simulink model "conicaltank"  (R2021a)
settings: Solver=ode45  StartTime=0.0  StopTime=30  RelTol=1e-3  EnableMultiTasking=on
settings Model: Creator=Administrator  LastModifiedBy=rakhul
settings SolverCC: AlgebraicLoopSolver=TrustRegion
settings DataIOCC: ExternalInput=[0 111.111]  InitialState=[]  LimitDataPoints=on  LoadExternalInput=on  LoadInitialState=on  SaveFormat=Array  ReturnWorkspaceOutputs=off
settings OptimizationCC: DefaultParameterBehavior=Inlined  BufferReuse=off  LifeSpan=inf
settings DebuggingCC: UnderspecifiedInitializationDetection=Classic  MergeDetectMultiDrivingBlocksExec=none  SolverPrmCheckMsg=warning  StateNameClashWarn=warning  InitInArrayFormatMsg=none  SFUnexpectedBacktrackingDiag=warning  SFNoUnconditionalDefaultTransitionDiag=warning  SFExecutionAtInitializationDiag=none  SFMachineParentedDataDiag=warning  ArithmeticOperatorsInVariantConditions=warning
settings HardwareCC: ProdBitPerPointer=32  ProdBitPerSizeT=32  ProdBitPerPtrDiffT=32  ProdLargestAtomicFloat=None  ProdIntDivRoundTo=Undefined  ProdEndianess=Unspecified  ProdWordSize=32  ProdHWDeviceType=32-bit Generic
settings ModelReferenceCC: PropagateSignalLabelsOutOfModel=off
settings SFSimCC: SimUseLocalCustomCode=off  CustomCodeUndefinedFunction=UseInterfaceOnly
settings RTWCC: RTWUseLocalCustomCode=off
settings CodeAppCC: StateflowObjectComments=on
settings GRTTargetCC: TargetLangStandard=C89/C90 (ANSI)
settings ConfigComp: CovMetricSettings=dw  CovSaveCumulativeToWorkspaceVar=on  CovSaveSingleToWorkspaceVar=on  CovExternalEMLEnable=off

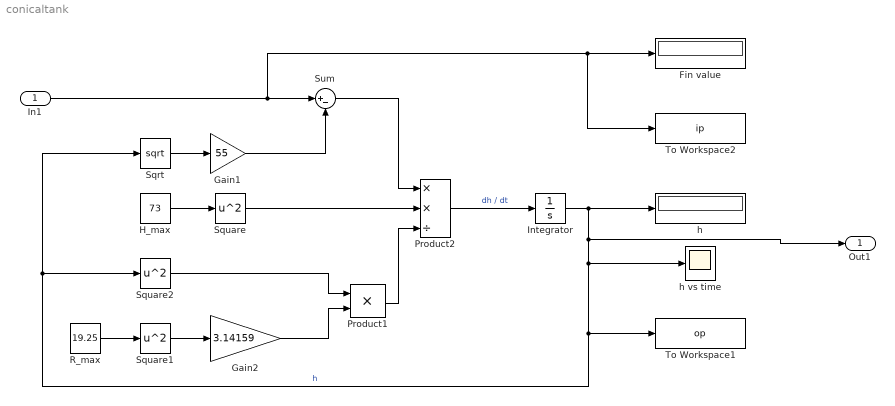
== system conicaltank ==
  In1 : Inport
  Fin value : Display
  Gain1 : Gain  Gain=55
  Gain2 : Gain  Gain=3.14159
  H_max : Constant  Value=73
  Integrator : Integrator  InitialCondition=2
  Product1 : Product  Inputs=**
  Product2 : Product  Inputs=**/
  R_max : Constant  Value=19.25
  Sqrt : Sqrt  SaturateOnIntegerOverflow=on
  Square : Math  Operator=square  SaturateOnIntegerOverflow=on
  Square1 : Math  Operator=square  SaturateOnIntegerOverflow=on
  Square2 : Math  Operator=square  SaturateOnIntegerOverflow=on
  Sum : Sum  Inputs=|+-
  To Workspace1 : ToWorkspace  VariableName=op  SampleTime=-1
  To Workspace2 : ToWorkspace  VariableName=ip  SampleTime=-1
  h : Display
  h vs time : Scope
  Out1 : Outport
  wires:
  Integrator/1 -> h/1, Out1/1, To Workspace1/1, Sqrt/1, Square2/1, h vs time/1  "h"
  Product2/1 -> Integrator/1  "dh / dt"
  Gain1/1 -> Sum/2
  Sum/1 -> Product2/1
  H_max/1 -> Square/1
  Product1/1 -> Product2/3
  Square/1 -> Product2/2
  Sqrt/1 -> Gain1/1
  R_max/1 -> Square1/1
  Square1/1 -> Gain2/1
  Square2/1 -> Product1/1
  Gain2/1 -> Product1/2
  In1/1 -> Sum/1, To Workspace2/1, Fin value/1
